simulink model "pc_linear_model"  (R2020a)
settings: Solver=VariableStepAuto  StartTime=0.0  StopTime=10  RelTol=1e-3
undefined symbols (not defined in the file or in its folder): A_hat, B_hat, C, k_d, Ts, x0
settings Model: Creator=mehdikoochak  LastModifiedBy=mehdikoochak

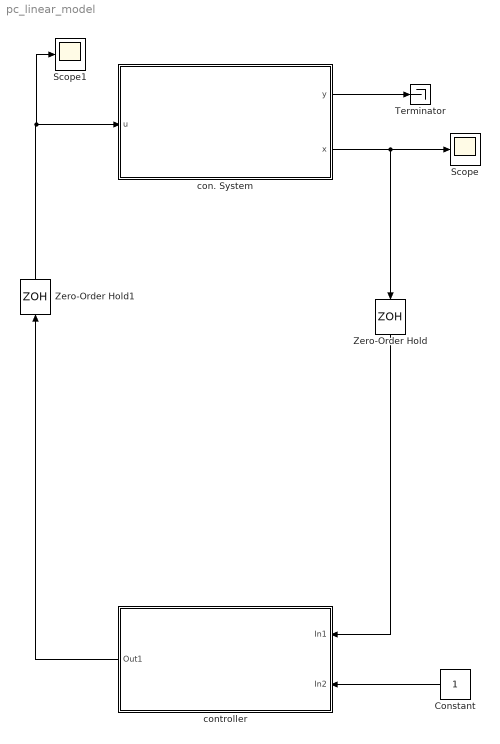
== system pc_linear_model ==
  Constant : Constant
  Scope : Scope
  Scope1 : Scope
  Terminator : Terminator
  Zero-Order Hold : ZeroOrderHold  SampleTime=Ts
  Zero-Order Hold1 : ZeroOrderHold  SampleTime=Ts
  con. System : Subsystem
  controller : Subsystem
  wires:
  con. System/1(y) -> Terminator/1
  con. System/2(x) -> Zero-Order Hold/1, Scope/1
  controller/1(Out1) -> Zero-Order Hold1/1
  Constant/1 -> controller/2(In2)
  Zero-Order Hold/1 -> controller/1(In1)
  Zero-Order Hold1/1 -> Scope1/1, con. System/1(u)

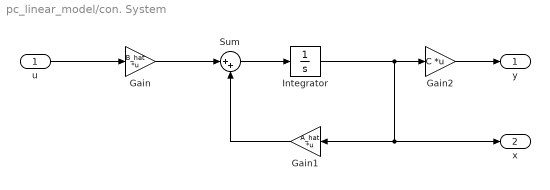
== system pc_linear_model/con. System ==
  u : Inport
  Gain : Gain  Gain=B_hat  Multiplication=Matrix(K*u)
  Gain1 : Gain  Gain=A_hat  Multiplication=Matrix(K*u)
  Gain2 : Gain  Gain=C  Multiplication=Matrix(K*u)
  Integrator : Integrator  InitialCondition=x0
  Sum : Sum  Inputs=|++
  y : Outport
  x : Outport  Port=2
  wires:
  Gain2/1 -> y/1
  Gain/1 -> Sum/1
  Sum/1 -> Integrator/1
  u/1 -> Gain/1
  Gain1/1 -> Sum/2
  Integrator/1 -> x/1, Gain1/1, Gain2/1

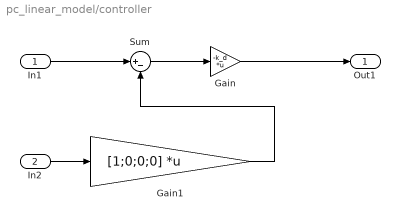
== system pc_linear_model/controller ==
  In1 : Inport
  In2 : Inport  Port=2
  Gain : Gain  Gain=-k_d  Multiplication=Matrix(K*u)
  Gain1 : Gain  Gain=[1;0;0;0]  Multiplication=Matrix(K*u)
  Sum : Sum  Inputs=|+-
  Out1 : Outport
  wires:
  Gain/1 -> Out1/1
  In1/1 -> Sum/1
  Sum/1 -> Gain/1
  In2/1 -> Gain1/1
  Gain1/1 -> Sum/2
